simulink model "storage"  (R2015b)
settings: Solver=VariableStepAuto  StartTime=0.0  StopTime=1  RelTol=1e-3
libraries: powerlib x38, powerlib_extras x6, powerlib_meascontrol x2
settings Model: Creator=fujitsu  LastModifiedBy=fujitsu

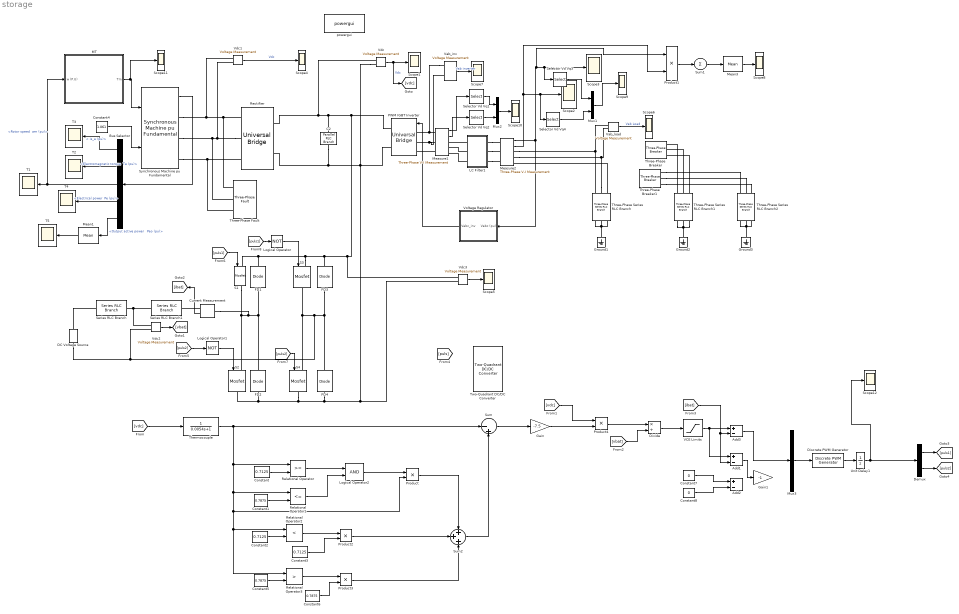
== system storage ==
  Add1 : Sum  Inputs=+-
  Add2 : Sum  Inputs=+-
  Add3 : Sum  Inputs=+-
  Bus Selector : BusSelector  OutputSignals="Stator current. is_a (pu),Mechanical.Electromagnetic torque  Te (pu),Mechanical.Rotor speed  wm (pu),Mechanical.Electrical power  Pe (pu),Output active power   Peo (pu)"
  C2 : powerlib/Elements/Parallel RLC Branch  LConnTagsString=a  RConnTagsString=__new0  BranchType=C  Resistance=inf  Inductance=inf  SetiL0=off  InitialCurrent=0  Capacitance=5000e-06  Setx0=off  InitialVoltage=0  Measurements=None
  Constant : Constant  Value=0.7125
  Constant1 : Constant  Value=0.7875
  Constant2 : Constant  Value=0.7125
  Constant3 : Constant  Value=0.7125
  Constant4 : Constant  Value=1.061
  Constant5 : Constant  Value=0.7875
  Constant6 : Constant  Value=0.7875
  Constant7 : Constant  Value=0
  Constant8 : Constant  Value=0
  Current Measurement : powerlib/Measurements/Current Measurement  PhasorSimulation=off  OutputType=Complex  PSBequivalent=0
  DC Voltage Source : powerlib/Electrical Sources/DC Voltage Source  Amplitude=800  Measurements=None
  Demux : Demux  Outputs=2
  Discrete PWM Generator : powerlib_extras/Discrete  Control Blocks/Discrete PWM Generator  GeneratorMode="1-arm  bridge (2 pulses)"  Fc=2000  Ts=5e-6  Internal=off  mIndex=0.4  Freq=60  Phase=0
  Divide : Product  Inputs=*/
  FD{1..4} (4 alike) : powerlib/Power Electronics/Diode  Ron=0.001  Lon=0  Vf=0.8  IC=0  UseSnubber=off  Rs=500  Cs=250e-9  Measurements=off
  Gain : Gain  Gain=-7.5
  Gain1 : Gain  Gain=-1
  Ground1 : powerlib/Elements/Ground  LConnTagsString=a
  Ground2 : powerlib/Elements/Ground  LConnTagsString=a
  Ground3 : powerlib/Elements/Ground  LConnTagsString=a
  LC Filter1 : Subsystem
  Logical Operator : Logic  Operator=NOT  AllPortsSameDT=off  OutDataTypeStr=boolean
  Logical Operator1 : Logic  Operator=NOT  AllPortsSameDT=off  OutDataTypeStr=boolean
  Logical Operator2 : Logic  AllPortsSameDT=off  OutDataTypeStr=boolean
  MT : Subsystem
  Mean1 : powerlib_meascontrol/Measurements/Mean  Freq=50  Vinit=0  Ts=50e-6
  Mean3 : powerlib_meascontrol/Measurements/Mean  Freq=50  Vinit=0  Ts=50e-6
  Measure1 : powerlib/Measurements/Three-Phase V-I Measurement  VoltageMeasurement=phase-to-phase  SetLabelV=off  LabelV=V1  Vpu=off  VpuLL=off  CurrentMeasurement=yes  SetLabelI=off  LabelI=I1  Ipu=off  Pbase=10e3  Vbase=400  OutputType=Magnitude  PhasorSimulation=off  PSBequivalent=0
  Measure2 : powerlib/Measurements/Three-Phase V-I Measurement  VoltageMeasurement=phase-to-phase  SetLabelV=off  LabelV=V1  Vpu=off  VpuLL=on  CurrentMeasurement=yes  SetLabelI=off  LabelI=I1  Ipu=on  Pbase=10e3  Vbase=400  OutputType=Magnitude  PhasorSimulation=off  PSBequivalent=0
  Mux1 : Mux  Inputs=2
  Mux2 : Mux  Inputs=2
  Mux3 : Mux  Inputs=1
  PWM IGBT Inverter : powerlib/Power Electronics/Universal Bridge  Arms=3  SnubberResistance=5000  SnubberCapacitance=inf  Device=IGBT / Diodes  Ron=1e-3  Lon=0  ForwardVoltages="[  0.0  0.0  ]"  ForwardVoltage=.8  GTOparameters=[ 1e-6 ,1e-6 ]  IGBTparameters=[ 1e-6 , 2e-6 ]  Measurements=Device currents  Measurements_2=None  converterType=Rectifier
  Product{,2..4} (4 alike) : Product
  Product1 : Product  SaturateOnIntegerOverflow=on  InputSameDT=on  OutDataTypeStr=Inherit: Same as first input
  Rectifier : powerlib/Power Electronics/Universal Bridge  Arms=3  SnubberResistance=50  SnubberCapacitance=0.1e-6  Device=Diodes  Ron=1e-3  Lon=0  ForwardVoltages="[  0.8  0.8  ]"  ForwardVoltage=.7  GTOparameters=[ 10e-6 , 20e-6 ]  IGBTparameters=[ 1e-6 , 2e-6 ]  Measurements=Device currents  Measurements_2=None  converterType=Rectifier
  Relational Operator : RelationalOperator  OutDataTypeStr=boolean
  Relational Operator1 : RelationalOperator  Operator=<=  OutDataTypeStr=boolean
  Relational Operator2 : RelationalOperator  Operator=<  OutDataTypeStr=boolean
  Relational Operator3 : RelationalOperator  Operator=>  OutDataTypeStr=boolean
  S{1..4} (4 alike) : powerlib/Power Electronics/Mosfet  Ron=0.1  Lon=0  Rd=0.01  Vfd=0  IC=0  Rs=1e5  Cs=inf  Measurements=off
  Scope{1..12} (12 alike) : Scope
  Selector Vd Vq{1..4} (4 alike) : Selector  InputPortWidth=3  IndexOptions=Index vector (dialog)  Indices=[1]  OutputSizes=1
  Series RLC Branch : powerlib/Elements/Series RLC Branch  LConnTagsString=__new0  RConnTagsString=__new0  BranchType=R  Resistance=0.0196  Inductance=1e-3  SetiL0=off  InitialCurrent=0  Capacitance=1e-6  Setx0=off  InitialVoltage=0  Measurements=None
  Series RLC Branch1 : powerlib/Elements/Series RLC Branch  LConnTagsString=__new0  RConnTagsString=__new0  BranchType=L  Resistance=0.0196  Inductance=0.004  SetiL0=off  InitialCurrent=0  Capacitance=1e-6  Setx0=off  InitialVoltage=0  Measurements=None
  Sum : Sum  Inputs=|-+
  Sum1 : Sum  Inputs=1  SaturateOnIntegerOverflow=on  InputSameDT=on  OutDataTypeStr=Inherit: Same as first input
  Sum2 : Sum  Inputs=+++
  Synchronous Machine pu Fundamental : powerlib/Machines/Synchronous Machine pu Fundamental  PresetModel=No  MechanicalLoad=Mechanical power Pm  ShowDetailedParameters=on  RotorType=Salient-pole  Units=per unit fundamental parameters  MeasurementBus=off  NominalParameters="[ 65e3  500 1500]"  Stator="[ 0.2503  0.114  0.6875  0.6875 ]"  Field="[ 1  10e15/(100*pi)]"  Dampers2=[0.0652, 0.5134, 0.0287, 0.2553, 7.765e-3, 0.9167 ]  Dampers1="[ 1.17E-02  0.182  1.97E-02  0.384 ]"  Mechanical=[ 6 0 2]  PolePairs=20  InitialConditions="[ 0  0  0  0  0  0  0  0  1 ]"  SetSaturation=off  Saturation=[0.6404,0.7127,0.8441,0.9214,0.9956,1.082,1.19,1.316,1.457;0.7,0.7698,0.8872,0.9466,0.9969,1.046,1.1,1.151,1.201]  LoadFlowParameters=[1,0,0,0,0]  TsPowergui=0  TsBlock=-1  IterativeModel=Trapezoidal non iterative  BusType=swing  Pref=0  Qref=0  Qmin=-inf  Qmax=inf  PLF=0  QLF=0
  T{1..5} (5 alike) : Scope
  Thermocouple : TransferFcn  Denominator="[0.0054  1]"
  Three-Phase Series RLC Branch : powerlib/Elements/Three-Phase Series RLC Branch  LConnTagsString=A|B|C  RConnTagsString=A|B|C  BranchType=R  Resistance=50  Inductance=1e-3  Capacitance=1e-6  Measurements=None
  Three-Phase Series RLC Branch1 : powerlib/Elements/Three-Phase Series RLC Branch  LConnTagsString=A|B|C  RConnTagsString=A|B|C  BranchType=R  Resistance=25  Inductance=1e-3  Capacitance=1e-6  Measurements=None
  Three-Phase Series RLC Branch2 : powerlib/Elements/Three-Phase Series RLC Branch  LConnTagsString=A|B|C  RConnTagsString=A|B|C  BranchType=R  Resistance=35  Inductance=1e-3  Capacitance=1e-6  Measurements=None
  Three-Phase Breaker : powerlib/Elements/Three-Phase Breaker  InitialState=closed  SwitchA=on  SwitchB=on  SwitchC=on  SwitchTimes=[10 20]  External=off  BreakerResistance=0.01  SnubberResistance=1e6  SnubberCapacitance=inf  Measurements=None
  Three-Phase Breaker1 : powerlib/Elements/Three-Phase Breaker  InitialState=open  SwitchA=on  SwitchB=on  SwitchC=on  SwitchTimes=[8 15]  External=off  BreakerResistance=0.01  SnubberResistance=1e6  SnubberCapacitance=inf  Measurements=None
  Three-Phase Fault : powerlib/Elements/Three-Phase Fault  InitialStates=0  FaultA=on  FaultB=on  FaultC=on  GroundFault=on  SwitchTimes=[0.3 0.6]  External=off  SwitchStatus=NaN  FaultResistance=0.001  GroundResistance=0.01  SnubberResistance=1e6  SnubberCapacitance=inf  Measurements=None
  Two-Quadrant DC/DC Converter : powerlib/Power Electronics/Two-Quadrant DC//DC Converter  ModelType=Switching devices  Ron=1e-3  Rs=1e6  Cs=inf  Vforward=[0,0]  Ron_Diode=1e-3  Rs_Diode=1e6  Cs_Diode=inf  Vf_Diode=1e-3  Rs_CurrentSource=inf
  Unit Delay1 : UnitDelay  SampleTime=2e-6
  VCE Limits : Saturate  UpperLimit=0.8  LowerLimit=-0.8
  Vab_inv : powerlib/Measurements/Voltage Measurement  Tag=PoWeRsYsTeMmEaSuReMeNt  PhasorSimulation=off  OutputType=Magnitude  PSBequivalent=0
  Vab_load : powerlib/Measurements/Voltage Measurement  Tag=PoWeRsYsTeMmEaSuReMeNt  PhasorSimulation=off  OutputType=Magnitude  PSBequivalent=0
  Vdc{,1..3} (4 alike) : powerlib/Measurements/Voltage Measurement  Tag=PoWeRsYsTeMmEaSuReMeNt  PhasorSimulation=off  OutputType=Magnitude  PSBequivalent=0
  Voltage Regulator : Subsystem  mask{kp=0.01, ki=5}
  powergui : powerlib/powergui  SimulationMode=Discrete  SolverType=Tustin  SampleTime=5e-6  frequency=60  SPID=off  DisableSnubberDevices=off  DisableRonSwitches=off  DisableVfSwitches=off  SwTol=0  DisplayEquations=off  Interpol=off  ExternalGateDelay=off  methode=off  Ts=0  FunctionMessages=off  echomessages=off  HookPort=off  EnableUseOfTLC=off  x0status=blocks  frequencyindice=0  Pbase=100e6  ErrMax=0.0001  Iterations=50  UnitsV=kV  UnitsW=MW  buscounter=0  RestoreLinks=warning  ResistiveCurrentMeasurement=off  Frange=[0:2:500]  Ylog=off  Xlog=on  ShowGrid=off  save=off  variable=ZData  structure=Vs  ZoomFFT=on  StartTime=1/60  cycles=1  DisplayStyle=1  fundamental=60  FreqAxis=on  MaxFrequency=10000  frequencyindicesteady=1  RmsSteady=1  display=off
  wires:
  Vdc/1 -> [vdc], Scope1/1  "Vdc"
  Vab_load/1 -> Scope6/1  "Vab Load"
  Vab_inv/1 -> Scope7/1  "Vab inverter"
  MT/1(Tm) -> Scope11/1, Synchronous Machine pu Fundamental/1
  Synchronous Machine pu Fundamental/1 -> Bus Selector/1
  Bus Selector/1 -> T3/1  "< is_a (pu)>"
  Bus Selector/2 -> T2/1  "<Electromagnetic torque  Te (pu)>"
  Bus Selector/3 -> MT/1(w (P.U)), T1/1  "<Rotor speed  wm (pu)>"
  Constant4/1 -> Synchronous Machine pu Fundamental/2
  Voltage Regulator/1(Vabc_inv) -> PWM IGBT Inverter/1
  Measure2/1 -> Product1/1, Selector Vd Vq3/1, Scope3/1, Voltage Regulator/1(Vabc (pu))
  Vdc1/1 -> Scope4/1  "Vdc"
  Bus Selector/4 -> T4/1  "<Electrical power  Pe (pu)>"
  Bus Selector/5 -> Mean1/1  "<Output active power   Peo (pu)>"
  Mean1/1 -> T5/1
  Measure2/2 -> Product1/2, Selector Vd Vq4/1, Scope2/1
  Mean3/1 -> Scope8/1
  Mux1/1 -> Scope9/1
  Mux2/1 -> Scope10/1
  Measure1/1 -> Selector Vd Vq1/1
  Selector Vd Vq1/1 -> Mux2/1
  Measure1/2 -> Selector Vd Vq2/1
  Selector Vd Vq2/1 -> Mux2/2
  Sum1/1 -> Mean3/1
  Product1/1 -> Sum1/1
  Selector Vd Vq3/1 -> Mux1/1
  Selector Vd Vq4/1 -> Mux1/2
  [vdc] -> Thermocouple/1
  Thermocouple/1 -> Sum/1, Relational Operator1/1, Product/2, Relational Operator2/1, Relational Operator3/1, Relational Operator/1
  Constant/1 -> Relational Operator/2
  Product/1 -> Sum2/1
  Constant1/1 -> Relational Operator1/2
  Relational Operator/1 -> Logical Operator2/1
  Relational Operator1/1 -> Logical Operator2/2
  Logical Operator2/1 -> Product/1
  Constant2/1 -> Relational Operator2/2
  Relational Operator2/1 -> Product2/1
  Constant3/1 -> Product2/2
  Product2/1 -> Sum2/2
  Constant5/1 -> Relational Operator3/2
  Relational Operator3/1 -> Product3/1
  Constant6/1 -> Product3/2
  Product3/1 -> Sum2/3
  Sum2/1 -> Sum/2
  Sum/1 -> Gain/1
  Gain/1 -> Product4/2
  [vdc] -> Product4/1
  Vdc2/1 -> [vbat]
  Product4/1 -> Divide/1
  [vbat] -> Divide/2
  Divide/1 -> VCE Limits/1
  VCE Limits/1 -> Add1/1, Add3/1
  Constant7/1 -> Add2/1
  Constant8/1 -> Add2/2
  Add3/1 -> Mux3/1
  Current Measurement/1 -> [ibat]
  [ibat] -> Add1/2, Add3/2
  Add1/1 -> Gain1/1
  Discrete PWM Generator/1 -> Unit Delay1/1
  Mux3/1 -> Discrete PWM Generator/1
  Unit Delay1/1 -> Scope12/1, Demux/1
  Logical Operator/1 -> S3/1
  Logical Operator1/1 -> S2/1
  Vdc3/1 -> Scope5/1
  Demux/1 -> [puls1]
  Demux/2 -> [puls2]
  [puls2] -> Logical Operator1/1
  [puls1] -> S1/1
  [puls2] -> S4/1
  [puls1] -> Logical Operator/1
  connections:
  Measure1/LConn2 -- PWM IGBT Inverter/LConn2 -- Vab_inv/LConn2
  Vab_inv/LConn1 -- PWM IGBT Inverter/LConn1 -- Measure1/LConn1
  Three-Phase Series RLC Branch/LConn1 -- Measure2/RConn1 -- Vab_load/LConn1
  Three-Phase Series RLC Branch/LConn2 -- Measure2/RConn2 -- Vab_load/LConn2
  Synchronous Machine pu Fundamental/RConn1 -- Vdc1/LConn1 -- Three-Phase Fault/LConn1 -- Rectifier/LConn1
  Rectifier/LConn2 -- Three-Phase Fault/LConn2 -- Synchronous Machine pu Fundamental/RConn2 -- Vdc1/LConn2
  Three-Phase Series RLC Branch/RConn2 -- Ground1/LConn1 -- Three-Phase Series RLC Branch/RConn3 -- Three-Phase Series RLC Branch/RConn1
  Three-Phase Series RLC Branch1/RConn2 -- Ground2/LConn1 -- Three-Phase Series RLC Branch1/RConn1 -- Three-Phase Series RLC Branch1/RConn3
  Three-Phase Series RLC Branch/LConn3 -- Measure2/RConn3
  Three-Phase Series RLC Branch2/RConn2 -- Ground3/LConn1 -- Three-Phase Series RLC Branch2/RConn1 -- Three-Phase Series RLC Branch2/RConn3
  Three-Phase Series RLC Branch1/LConn1 -- Three-Phase Breaker/RConn1
  Three-Phase Series RLC Branch1/LConn2 -- Three-Phase Breaker/RConn2
  Three-Phase Series RLC Branch1/LConn3 -- Three-Phase Breaker/RConn3
  Synchronous Machine pu Fundamental/RConn3 -- Three-Phase Fault/LConn3 -- Rectifier/LConn3
  Measure1/LConn3 -- PWM IGBT Inverter/LConn3
  LC Filter1/RConn1 -- Measure2/LConn1
  LC Filter1/RConn2 -- Measure2/LConn2
  LC Filter1/RConn3 -- Measure2/LConn3
  LC Filter1/LConn1 -- Measure1/RConn1
  LC Filter1/LConn2 -- Measure1/RConn2
  LC Filter1/LConn3 -- Measure1/RConn3
  Three-Phase Breaker1/RConn1 -- Three-Phase Series RLC Branch2/LConn1
  Three-Phase Breaker1/RConn2 -- Three-Phase Series RLC Branch2/LConn2
  Three-Phase Breaker1/RConn3 -- Three-Phase Series RLC Branch2/LConn3
  Series RLC Branch/LConn1 -- DC Voltage Source/RConn1
  Series RLC Branch1/LConn1 -- Vdc2/LConn1 -- Series RLC Branch/RConn1
  FD2/RConn1 -- FD1/LConn1 -- Current Measurement/LConn1 -- S1/RConn1 -- S2/LConn1
  Current Measurement/RConn1 -- Series RLC Branch1/RConn1
  S3/LConn1 -- Vdc3/LConn1 -- PWM IGBT Inverter/RConn1 -- Vdc/LConn1 -- Rectifier/RConn1 -- C2/LConn1 -- FD3/RConn1 -- FD1/RConn1 -- S1/LConn1
  DC Voltage Source/LConn1 -- S3/RConn1 -- S4/LConn1 -- FD4/RConn1 -- FD3/LConn1 -- Vdc2/LConn2
  Vdc/LConn2 -- C2/RConn1 -- Rectifier/RConn2 -- FD2/LConn1 -- S2/RConn1 -- S4/RConn1 -- FD4/LConn1 -- Vdc3/LConn2 -- PWM IGBT Inverter/RConn2

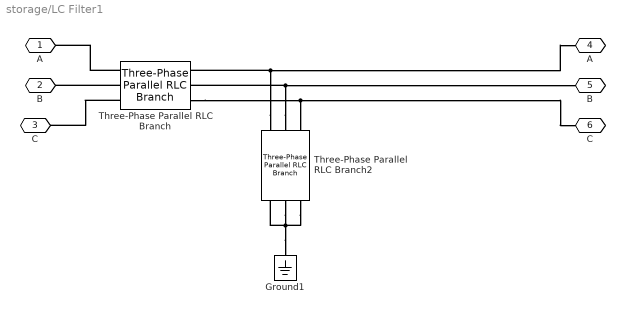
== system storage/LC Filter1 ==
  Ground1 : powerlib/Elements/Ground  LConnTagsString=a
  Three-Phase Parallel RLC Branch : powerlib/Elements/Three-Phase Parallel RLC Branch  LConnTagsString=A|B|C  RConnTagsString=A|B|C  BranchType=L  Resistance=1  Inductance=5.7e-3  Capacitance=1e-6  Measurements=None
  Three-Phase Parallel RLC Branch2 : powerlib/Elements/Three-Phase Parallel RLC Branch  LConnTagsString=A|B|C  RConnTagsString=A|B|C  BranchType=C  Resistance=1  Inductance=5.7e-3  Capacitance=1000e-6  Measurements=None
  A : PMIOPort  Port=1  Side=Left
  B : PMIOPort  Port=2  Side=Left
  C : PMIOPort  Port=3  Side=Left
  "A " : PMIOPort  Port=4  Side=Right
  "B " : PMIOPort  Port=5  Side=Right
  "C " : PMIOPort  Port=6  Side=Right
  connections:
  Ground1/LConn1 -- Three-Phase Parallel RLC Branch2/RConn2 -- Three-Phase Parallel RLC Branch2/RConn1 -- Three-Phase Parallel RLC Branch2/RConn3
  Three-Phase Parallel RLC Branch/RConn3 -- Three-Phase Parallel RLC Branch2/LConn3 -- "C "/RConn1
  Three-Phase Parallel RLC Branch2/LConn2 -- "B "/RConn1 -- Three-Phase Parallel RLC Branch/RConn2
  Three-Phase Parallel RLC Branch2/LConn1 -- "A "/RConn1 -- Three-Phase Parallel RLC Branch/RConn1
  Three-Phase Parallel RLC Branch/LConn3 -- C/RConn1
  Three-Phase Parallel RLC Branch/LConn2 -- B/RConn1
  Three-Phase Parallel RLC Branch/LConn1 -- A/RConn1

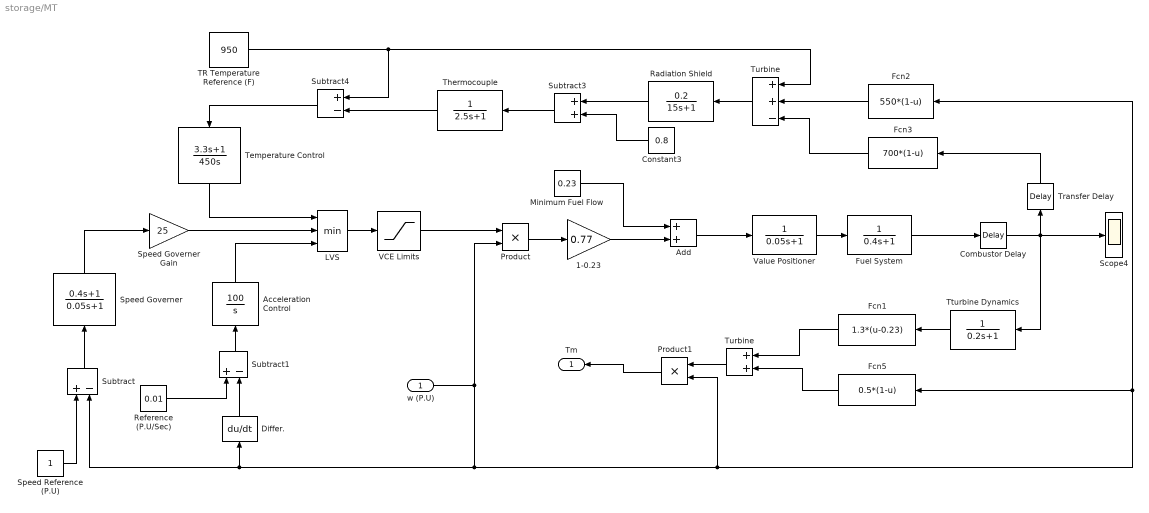
== system storage/MT ==
  w (P.U) : Inport
  1-0.23 : Gain  Gain=0.77
  Acceleration Control : TransferFcn  Numerator=[0 100]  Denominator=[1 0]
  Add : Sum
  Combustor Delay : TransportDelay  DelayTime=0.01
  Constant3 : Constant  Value=0.8
  Differ. : Derivative
  Fcn1 : Fcn  Expr=1.3*(u-0.23)
  Fcn2 : Fcn  Expr=550*(1-u)
  Fcn3 : Fcn  Expr=700*(1-u)
  Fcn5 : Fcn  Expr=0.5*(1-u)
  Fuel System : TransferFcn  Denominator=[0.4 1]
  LVS : MinMax  Inputs=3
  Minimum Fuel Flow : Constant  Value=0.23
  Product : Product  RndMeth=Zero
  Product1 : Product  RndMeth=Zero
  Radiation Shield : TransferFcn  Numerator=[0.2]  Denominator=[15 1]
  Reference (P.U/Sec) : Constant  Value=0.01
  Scope4 : Scope
  Speed Governer : TransferFcn  Numerator=[0.4 1]  Denominator=[0.05 1]
  Speed Governer Gain : Gain  Gain=25
  Speed Reference (P.U) : Constant
  Subtract : Sum  Inputs=+-
  Subtract1 : Sum  Inputs=+-
  Subtract3 : Sum
  Subtract4 : Sum  Inputs=+-
  TR Temperature Reference (F) : Constant  Value=950
  Temperature Control : TransferFcn  Numerator=[3.3 1]  Denominator=[450 0]
  Thermocouple : TransferFcn  Denominator=[2.5 1]
  Transfer Delay : TransportDelay  DelayTime=0.04
  Tturbine Dynamics : TransferFcn  Denominator=[0.2 1]
  Turbine : Sum  Inputs=++-
  "Turbine " : Sum
  VCE Limits : Saturate  UpperLimit=1.5  LowerLimit=-0.1
  Value Positioner : TransferFcn  Denominator=[0.05 1]
  Tm : Outport
  wires:
  Speed Reference (P.U)/1 -> Subtract/1
  Subtract/1 -> Speed Governer/1
  VCE Limits/1 -> Product/1
  Product/1 -> 1-0.23/1
  1-0.23/1 -> Add/2
  Minimum Fuel Flow/1 -> Add/1
  Add/1 -> Value Positioner/1
  Value Positioner/1 -> Fuel System/1
  Fuel System/1 -> Combustor Delay/1
  Combustor Delay/1 -> Tturbine Dynamics/1, Scope4/1, Transfer Delay/1
  Speed Governer Gain/1 -> LVS/2
  Differ./1 -> Subtract1/2
  Reference (P.U/Sec)/1 -> Subtract1/1
  Subtract1/1 -> Acceleration Control/1
  Acceleration Control/1 -> LVS/3
  LVS/1 -> VCE Limits/1
  Transfer Delay/1 -> Fcn3/1
  Fcn3/1 -> Turbine/3
  Fcn2/1 -> Turbine/2
  Radiation Shield/1 -> Subtract3/1
  Constant3/1 -> Subtract3/2
  Turbine/1 -> Radiation Shield/1
  Subtract3/1 -> Thermocouple/1
  Thermocouple/1 -> Subtract4/2
  TR Temperature Reference (F)/1 -> Turbine/1, Subtract4/1
  Subtract4/1 -> Temperature Control/1
  Temperature Control/1 -> LVS/1
  Speed Governer/1 -> Speed Governer Gain/1
  w (P.U)/1 -> Product/2, Subtract/2, Differ./1, Product1/2, Fcn5/1, Fcn2/1
  Tturbine Dynamics/1 -> Fcn1/1
  Fcn1/1 -> "Turbine "/1
  Fcn5/1 -> "Turbine "/2
  "Turbine "/1 -> Product1/1
  Product1/1 -> Tm/1

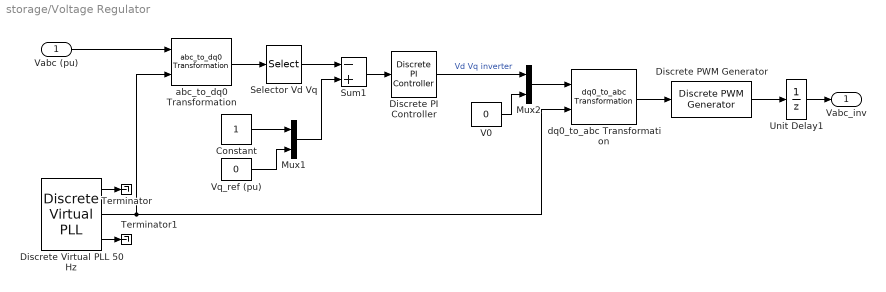
== system storage/Voltage Regulator ==
  Vabc (pu) : Inport
  Constant : Constant
  Discrete PI Controller : powerlib_extras/Discrete  Control Blocks/Discrete PI Controller  Kp=kp  Ki=ki  Par_Limits=[1 -1]  Init=0  Ts=5e-6
  Discrete PWM Generator : powerlib_extras/Discrete  Control Blocks/Discrete PWM Generator  GeneratorMode="3-arm  bridge (6 pulses)"  Fc=2000  Ts=5e-6  Internal=off  mIndex=0.4  Freq=60  Phase=0
  Discrete Virtual PLL 50 Hz : powerlib_extras/Discrete  Control Blocks/Discrete Virtual PLL  Freq=50  Phase=0  Ts=5e-6
  Mux1 : Mux  Inputs=2
  Mux2 : Mux  Inputs=2
  Selector Vd Vq : Selector  InputPortWidth=3  IndexOptions=Index vector (dialog)  Indices=[1 2]  OutputSizes=1
  Sum1 : Sum  Inputs=-+  SaturateOnIntegerOverflow=on  InputSameDT=on  OutDataTypeStr=Inherit: Same as first input
  Terminator : Terminator
  Terminator1 : Terminator
  Unit Delay1 : UnitDelay  SampleTime=2e-6
  V0 : Constant  Value=0
  Vq_ref (pu) : Constant  Value=0
  abc_to_dq0 Transformation : powerlib_extras/Measurements/abc_to_dq0 Transformation
  dq0_to_abc Transformation : powerlib_extras/Measurements/dq0_to_abc Transformation
  Vabc_inv : Outport
  wires:
  abc_to_dq0 Transformation/1 -> Selector Vd Vq/1
  Vabc (pu)/1 -> abc_to_dq0 Transformation/1
  Selector Vd Vq/1 -> Sum1/1
  Sum1/1 -> Discrete PI Controller/1
  Mux2/1 -> dq0_to_abc Transformation/1
  V0/1 -> Mux2/2
  Discrete Virtual PLL 50 Hz/2 -> abc_to_dq0 Transformation/2, dq0_to_abc Transformation/2
  Constant/1 -> Mux1/1
  Vq_ref (pu)/1 -> Mux1/2
  Mux1/1 -> Sum1/2
  Discrete Virtual PLL 50 Hz/1 -> Terminator/1
  Discrete Virtual PLL 50 Hz/3 -> Terminator1/1
  Discrete PI Controller/1 -> Mux2/1  "Vd Vq inverter"
  Discrete PWM Generator/1 -> Unit Delay1/1
  dq0_to_abc Transformation/1 -> Discrete PWM Generator/1
  Unit Delay1/1 -> Vabc_inv/1
